simulink model "Two_Input_Model_CO"  (R2021a)
settings: Solver=VariableStepAuto  StartTime=0.0  StopTime=10  RelTol=1e-3
values from neighbouring files (symbols this model uses):
  A = [0 0 0 0 0 0 0 0 0 -0.534142885228 22.5045950602 -13.9882516442 ... (36 elements, 6x6)]    [Values_Rev3.mat]
  B = [0 0 0 0.425188099574 -0.174236211288 -0.288671680413 0 0 0 -0.174236211288 7.34094843962 -4.56293631615 ... (18 elements, 6x3)]    [Values_Rev3.mat]
  C = [1 0 0 0 1 0 0 0 1 0 0 0 ... (18 elements, 3x6)]    [Values_Rev3.mat]
undefined symbols (not defined in the file or in its folder): K, L, v, x0
libraries: vrlib x2, aerolibanimutils x1, dspvision x1
settings Model: Creator=J44381  LastModifiedBy=vicen
settings SolverCC: AlgebraicLoopSolver=TrustRegion
settings DebuggingCC: SFMachineParentedDataDiag=warning

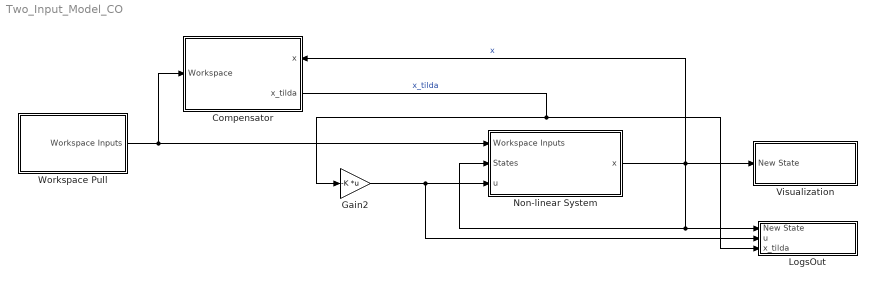
== system Two_Input_Model_CO ==
  Compensator : Subsystem
      settings: PortSchema="{\"entries\":[{\"content\":{\"sides\":[{\"content\":{\"connectorIds\":[\"In1\"]},\"type\":\"ConnectorPlacement.EquallySpacedRectSide\",\"uuid\":\"fa5a8305-86ae-432c-9810-dcf02cae709e\"},{\"content\":{\"connectorIds\":[\"In2\",\"Out1\"],\"side\":\"RIGHT\"},\"type\":\"ConnectorPlacement.EquallySpacedRectSide\",\"uuid\":\"5b9e218f-8372-497e-90c9-36ba94e4ea20\"},{\"content\":{\"connectorIds\":[],\"side\":\"TOP\"},\"type\":\"ConnectorPlacement.EquallySpacedRectSide\",\"uuid\":\"bf766896-0790-4646-8f59-54f411e82d6d\"}]},\"type\":\"ConnectorPlacement.EquallySpacedConnector\",\"uuid\":\"810fb74e-5609-4dc4-a3e8-0485af32c7e5\"}],\"packageUris\":[\"http://schema.mathworks.com/mf0/Connector/R2020b\"],\"version\":\"1.0\"}"
  Gain2 : Gain  Gain=-K  Multiplication=Matrix(K*u)
  LogsOut : Subsystem
  Non-linear System : Subsystem
  Visualization : Subsystem
  Workspace Pull : Subsystem
  wires:
  Workspace Pull/1("Workspace Inputs ") -> Compensator/1(Workspace), Non-linear System/1("Workspace Inputs ")
  Non-linear System/1(x) -> Compensator/2(x), Visualization/1(New State), Non-linear System/2(States), LogsOut/1(New State)  "x"
  Compensator/1(x_tilda) -> Gain2/1, LogsOut/3(x_tilda)  "x_tilda"
  Gain2/1 -> Non-linear System/3(u), LogsOut/2(u)

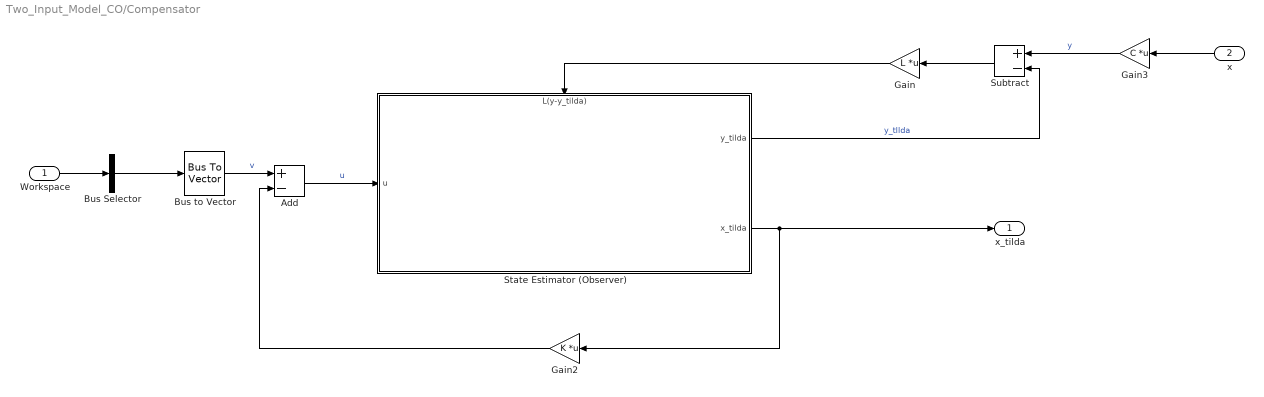
== system Two_Input_Model_CO/Compensator ==
  Workspace : Inport
  x : Inport  Port=2
  Add : Sum  Inputs=+-
  Bus Selector : BusSelector  OutputSignals=Reference_Signal  OutputAsBus=on
  Bus to Vector : BusToVector
  Gain : Gain  Gain=L  Multiplication=Matrix(K*u)
  Gain2 : Gain  Gain=K  Multiplication=Matrix(K*u)
  Gain3 : Gain  Gain=C  Multiplication=Matrix(K*u)
  State Estimator (Observer) : Subsystem
      settings: PortSchema="{\"entries\":[{\"content\":{\"sides\":[{\"content\":{\"connectorIds\":[\"In1\"]},\"type\":\"ConnectorPlacement.EquallySpacedRectSide\",\"uuid\":\"af437ed9-8515-47ce-9bf3-57578eb1cf2e\"},{\"content\":{\"connectorIds\":[\"Out1\",\"Out2\"],\"side\":\"RIGHT\"},\"type\":\"ConnectorPlacement.EquallySpacedRectSide\",\"uuid\":\"1ea6d729-9487-4493-ae4f-2f3f5c430ca0\"},{\"content\":{\"connectorIds\":[\"In2\"],\"side\":\"TOP\"},\"type\":\"ConnectorPlacement.EquallySpacedRectSide\",\"uuid\":\"e9fc0f2c-a064-4175-9528-0d44140d355b\"}]},\"type\":\"ConnectorPlacement.EquallySpacedConnector\",\"uuid\":\"af498723-3483-4ae8-9449-73d3fe9ce68c\"}],\"packageUris\":[\"http://schema.mathworks.com/mf0/Connector/R2020b\"],\"version\":\"1.0\"}"
  Subtract : Sum  Inputs=+-
  x_tilda : Outport
  wires:
  Add/1 -> State Estimator (Observer)/1(u)  "u"
  State Estimator (Observer)/1(y_tilda) -> Subtract/2  "y_tllda"
  Subtract/1 -> Gain/1
  Workspace/1 -> Bus Selector/1
  Bus Selector/1 -> Bus to Vector/1
  Bus to Vector/1 -> Add/1  "v"
  State Estimator (Observer)/2(x_tilda) -> Gain2/1, x_tilda/1
  Gain/1 -> State Estimator (Observer)/2(L(y-y_tilda))
  x/1 -> Gain3/1
  Gain2/1 -> Add/2
  Gain3/1 -> Subtract/1  "y"

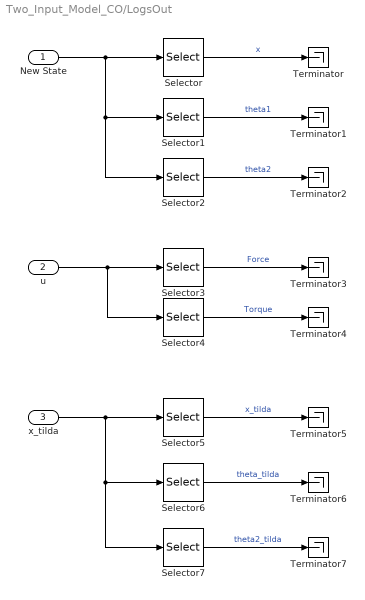
== system Two_Input_Model_CO/LogsOut ==
  New State : Inport
  u : Inport  Port=2
  x_tilda : Inport  Port=3
  Selector : Selector  InputPortWidth=6  IndexOptions=Index vector (dialog)  Indices=1  OutputSizes=1
  Selector1 : Selector  InputPortWidth=6  IndexOptions=Index vector (dialog)  Indices=2  OutputSizes=1
  Selector2 : Selector  InputPortWidth=6  IndexOptions=Index vector (dialog)  Indices=3  OutputSizes=1
  Selector3 : Selector  InputPortWidth=2  IndexOptions=Index vector (dialog)  Indices=1  OutputSizes=1
  Selector4 : Selector  InputPortWidth=2  IndexOptions=Index vector (dialog)  Indices=2  OutputSizes=1
  Selector5 : Selector  InputPortWidth=6  IndexOptions=Index vector (dialog)  Indices=1  OutputSizes=1
  Selector6 : Selector  InputPortWidth=6  IndexOptions=Index vector (dialog)  Indices=2  OutputSizes=1
  Selector7 : Selector  InputPortWidth=6  IndexOptions=Index vector (dialog)  Indices=3  OutputSizes=1
  Terminator{,1..7} (8 alike) : Terminator
  wires:
  Selector/1 -> Terminator/1  "x"
  Selector1/1 -> Terminator1/1  "theta1"
  Selector2/1 -> Terminator2/1  "theta2"
  New State/1 -> Selector2/1, Selector1/1, Selector/1
  u/1 -> Selector4/1, Selector3/1
  Selector4/1 -> Terminator4/1  "Torque"
  Selector3/1 -> Terminator3/1  "Force"
  x_tilda/1 -> Selector5/1, Selector7/1, Selector6/1
  Selector5/1 -> Terminator5/1  "x_tilda"
  Selector6/1 -> Terminator6/1  "theta_tilda"
  Selector7/1 -> Terminator7/1  "theta2_tilda"

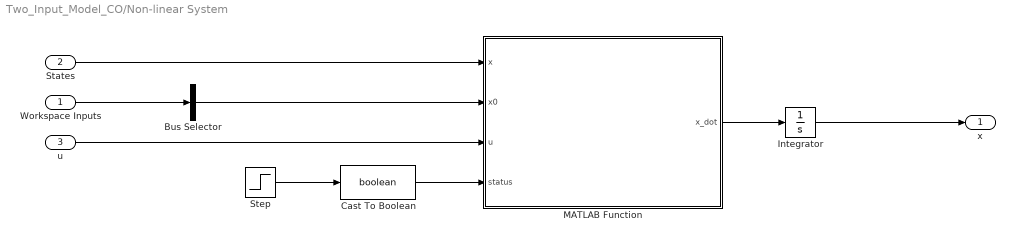
== system Two_Input_Model_CO/Non-linear System ==
  "Workspace Inputs " : Inport
  States : Inport  Port=2
  u : Inport  Port=3
  Bus Selector : BusSelector  OutputSignals=Initial_States  OutputAsBus=on
  Cast To Boolean : DataTypeConversion  OutDataTypeStr=boolean
  Integrator : Integrator  InitialCondition=[x0.x;x0.theta1;x0.theta2;x0.x_dot;x0.theta1_dot;x0.theta2_dot]
  MATLAB Function : MATLAB Function  TreatAsAtomicUnit=on
  Step : Step  Time=.01  SampleTime=0
  x : Outport
  wires:
  MATLAB Function/1(x_dot) -> Integrator/1
  States/1 -> MATLAB Function/1(x)
  "Workspace Inputs "/1 -> Bus Selector/1
  u/1 -> MATLAB Function/3(u)
  Bus Selector/1 -> MATLAB Function/2(x0)
  Integrator/1 -> x/1
  Step/1 -> Cast To Boolean/1
  Cast To Boolean/1 -> MATLAB Function/4(status)

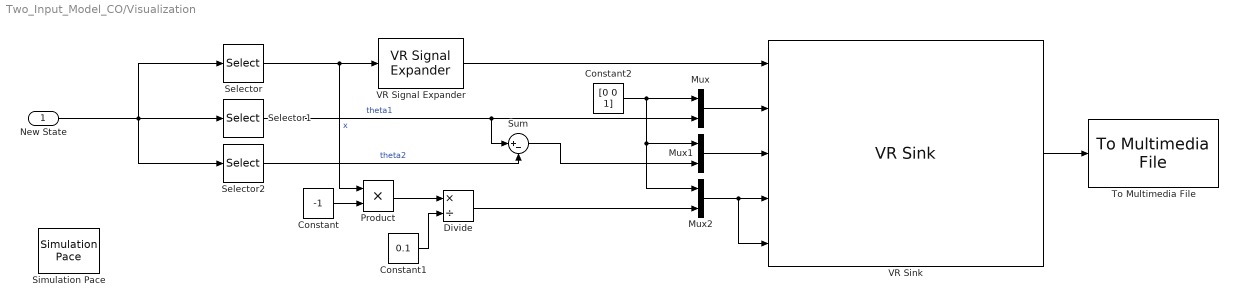
== system Two_Input_Model_CO/Visualization ==
  New State : Inport
  Constant : Constant  Value=-1
  Constant1 : Constant  Value=0.1
  Constant2 : Constant  Value=[0 0 1]
  Divide : Product  Inputs=*/
  Mux : Mux  Inputs=2
  Mux1 : Mux  Inputs=2
  Mux2 : Mux  Inputs=2
  Product : Product
  Selector : Selector  InputPortWidth=6  IndexOptions=Index vector (dialog)  Indices=1  OutputSizes=1
  Selector1 : Selector  InputPortWidth=6  IndexOptions=Index vector (dialog)  Indices=2  OutputSizes=1
  Selector2 : Selector  InputPortWidth=6  IndexOptions=Index vector (dialog)  Indices=3  OutputSizes=1
  Simulation Pace : aerolibanimutils/Simulation Pace  SimulationPace=1  SleepMode=Auto  OutputPaceError=off  SampleTime=1/30
  Sum : Sum  Inputs=|+-
  To Multimedia File : dspvision/To Multimedia File  outputFilename=output2.avi  streamSelection=Video only  videoCompressor=None (uncompressed)  audioCompressor=None (uncompressed)  imagePorts=One multidimensional signal  fileType=AVI  audioDatatype=Determine from input data type  fourcc=RGB  videoQuality=75  mj2000CompFactor=10
  VR Signal Expander : vrlib/VR Signal Expander  outwidth=3  outidx=[1]
  VR Sink : vrlib/VR Sink  InstantiateOnLoad=on  SampleTime=0.1  ViewEnable=on  RemoteChange=off  RemoteView=off  FieldsWritten=Cart.translation.3.1.1.double#Rotation1.rotation.4.1.1.double#Rotation2.rotation.4.1.1.double#Axis_Rotate.rotation.4.1.1.double#Axis_Rotate2.rotation.4.1.1.double  WorldFileName=Cart_Actual.WRL  AutoView=off  VideoDimensions=[1500 2000]  AllowVariableSize=off  FigureProperties="{'Position', 'Name', 'Viewpoint', 'CameraBound', 'CameraDirection', 'CameraPosition', 'CameraUpVector', 'ZoomFactor', 'Antialiasing', 'Headlight', 'Lighting', 'NavPanel', 'Sound', 'StatusBar', 'Stereo3D', 'Stereo3DCameraOffset', 'Stereo3DHIT', 'ToolBar', 'Textures', 'Transparency', 'Triad', 'Wireframe', 'NavZones', 'NavMode', 'NavSpeed', 'CaptureFileFormat', 'CaptureFileName', 'Record2DCompressMethod', 'Record2DCompressQuality', 'Record2D', 'Record2DFileName', 'Record2DFPS'; [1.2660000000000001e+02   9.4799999999999955e+01   8.0000000000000000e+02   6.0020000000000005e+02], '', '_untitled_1', 'on', [0.0000000000000000e+00   0.0000000000000000e+00  -1.0000000000000000e+00], [0.0000000000000000e+00   0.0000000000000000e+00   0.0000000000000000e+00], [0.0000000000000000e+00   1.0000000000000000e+00   0.0000000000000000e+00], [1.0000000000000000e+00], 'on', 'on', 'on', 'none', 'on', 'off', 'off', [1.0000000149011612e-01], [0.0000000000000000e+00], 'off', 'on', 'on', 'none', 'off', 'off', 'fly', 'normal', 'tif', '%f_anim_%n.tif', 'auto', [7.5000000000000000e+01], 'off', '***video***', 'auto'}"
  wires:
  New State/1 -> Selector/1, Selector2/1, Selector1/1
  Selector/1 -> VR Signal Expander/1, Product/1  "x"
  Selector1/1 -> Sum/1, Mux/2  "theta1"
  Product/1 -> Divide/1
  Constant/1 -> Product/2
  Constant1/1 -> Divide/2
  Constant2/1 -> Mux1/1, Mux2/1, Mux/1
  Selector2/1 -> Sum/2  "theta2"
  Divide/1 -> Mux2/2
  Sum/1 -> Mux1/2
  VR Signal Expander/1 -> VR Sink/1
  Mux/1 -> VR Sink/2
  Mux1/1 -> VR Sink/3
  Mux2/1 -> VR Sink/4, VR Sink/5
  VR Sink/1 -> To Multimedia File/1

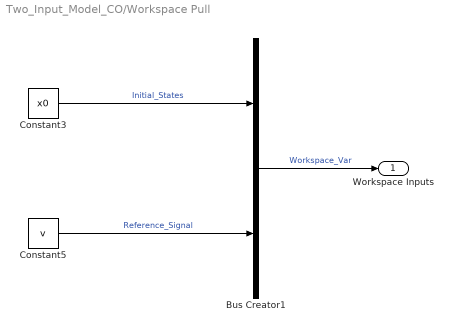
== system Two_Input_Model_CO/Workspace Pull ==
  Bus Creator1 : BusCreator  Inputs=2
  Constant3 : Constant  Value=x0  VectorParams1D=off  OutDataTypeStr=Bus: State_bus
  Constant5 : Constant  Value=v  VectorParams1D=off  OutDataTypeStr=Bus: Reference_bus
  "Workspace Inputs " : Outport
  wires:
  Bus Creator1/1 -> "Workspace Inputs "/1  "Workspace_Var"
  Constant3/1 -> Bus Creator1/1  "Initial_States"
  Constant5/1 -> Bus Creator1/2  "Reference_Signal"

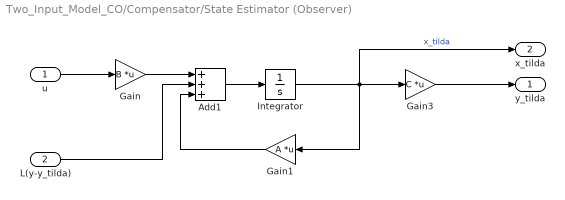
== system Two_Input_Model_CO/Compensator/State Estimator (Observer) ==
  u : Inport
  L(y-y_tilda) : Inport  Port=2
  Add1 : Sum  Inputs=+++
  Gain : Gain  Gain=B  Multiplication=Matrix(K*u)
  Gain1 : Gain  Gain=A  Multiplication=Matrix(K*u)
  Gain3 : Gain  Gain=C  Multiplication=Matrix(K*u)
  Integrator : Integrator  InitialCondition=[x0.x;0;0;x0.x_dot;x0.theta1_dot;x0.theta2_dot]
  y_tilda : Outport
  x_tilda : Outport  Port=2
  wires:
  Gain1/1 -> Add1/3
  Integrator/1 -> Gain3/1, x_tilda/1, Gain1/1  "x_tilda"
  Add1/1 -> Integrator/1
  Gain/1 -> Add1/1
  u/1 -> Gain/1
  Gain3/1 -> y_tilda/1
  L(y-y_tilda)/1 -> Add1/2

== matlab function Two_Input_Model_CO/Non-linear System/MATLAB Function ==
  data: x input; x0 input; u input; x_dot output; status input
function x_dot  = Nonlinear_Dynamics(x,x0,u,status)
    if status == false
        x2 = x0.theta1;
        x3 = x0.theta2;
        x4 = x0.x_dot;
        x5 = x0.theta1_dot;
        x6 = x0.theta2_dot;
        u1 = u(1);
        u2 = u(2);
    else
        x2 = x(2);
        x3 = x(3);
        x4 = x(4);
        x5 = x(5);
        x6 = x(6);
        u1 = u(1);
        u2 = u(2);
    end
    % Insert Equations
    x_dot = double([
                x4;
                x5;
                x6;
                x5*((15*x5*sin(x2 - x3)*(cos(x3) - cos(x2 - x3)*cos(x2)))/(2*(25*cos(x2)^2 + 15*cos(x3)^2 + 33*cos(x2 - x3)^2 - 30*cos(x2 - x3)*cos(x2)*cos(x3) - 55)) + (5*x5*sin(x2)*(3*cos(x2 - x3)^2 - 5))/(2*(25*cos(x2)^2 + 15*cos(x3)^2 + 33*cos(x2 - x3)^2 - 30*cos(x2 - x3)*cos(x2)*cos(x3) - 55))) - x6*((9*x6*sin(x2 - x3)*(5*cos(x2) - 3*cos(x2 - x3)*cos(x3)))/(4*(25*cos(x2)^2 + 15*cos(x3)^2 + 33*cos(x2 - x3)^2 - 30*cos(x2 - x3)*cos(x2)*cos(x3) - 55)) - (9*x6*sin(x3)*(3*cos(x2 - x3)^2 - 5))/(4*(25*cos(x2)^2 + 15*cos(x3)^2 + 33*cos(x2 - x3)^2 - 30*cos(x2 - x3)*cos(x2)*cos(x3) - 55))) + (981*sin(x2)*(5*cos(x2) - 3*cos(x2 - x3)*cos(x3)))/(20*(25*cos(x2)^2 + 15*cos(x3)^2 + 33*cos(x2 - x3)^2 - 30*cos(x2 - x3)*cos(x2)*cos(x3) - 55)) + (8*u2*(5*cos(x2) - 3*cos(x2 - x3)*cos(x3)))/(25*cos(x2)^2 + 15*cos(x3)^2 + 33*cos(x2 - x3)^2 - 30*cos(x2 - x3)*cos(x2)*cos(x3) - 55) + (2943*sin(x3)*(cos(x3) - cos(x2 - x3)*cos(x2)))/(20*(25*cos(x2)^2 + 15*cos(x3)^2 + 33*cos(x2 - x3)^2 - 30*cos(x2 - x3)*cos(x2)*cos(x3) - 55)) + (4*u1*(3*cos(x2 - x3)^2 - 5))/(25*cos(x2)^2 + 15*cos(x3)^2 + 33*cos(x2 - x3)^2 - 30*cos(x2 - x3)*cos(x2)*cos(x3) - 55);
                x5*((5*x5*sin(x2)*(5*cos(x2) - 3*cos(x2 - x3)*cos(x3)))/(25*cos(x2)^2 + 15*cos(x3)^2 + 33*cos(x2 - x3)^2 - 30*cos(x2 - x3)*cos(x2)*cos(x3) - 55) + (3*x5*sin(x2 - x3)*(11*cos(x2 - x3) - 5*cos(x2)*cos(x3)))/(25*cos(x2)^2 + 15*cos(x3)^2 + 33*cos(x2 - x3)^2 - 30*cos(x2 - x3)*cos(x2)*cos(x3) - 55)) + x6*((9*x6*sin(x3)*(5*cos(x2) - 3*cos(x2 - x3)*cos(x3)))/(2*(25*cos(x2)^2 + 15*cos(x3)^2 + 33*cos(x2 - x3)^2 - 30*cos(x2 - x3)*cos(x2)*cos(x3) - 55)) - (9*x6*sin(x2 - x3)*(3*cos(x3)^2 - 11))/(2*(25*cos(x2)^2 + 15*cos(x3)^2 + 33*cos(x2 - x3)^2 - 30*cos(x2 - x3)*cos(x2)*cos(x3) - 55))) + (2943*sin(x3)*(11*cos(x2 - x3) - 5*cos(x2)*cos(x3)))/(50*(25*cos(x2)^2 + 15*cos(x3)^2 + 33*cos(x2 - x3)^2 - 30*cos(x2 - x3)*cos(x2)*cos(x3) - 55)) + (981*sin(x2)*(3*cos(x3)^2 - 11))/(10*(25*cos(x2)^2 + 15*cos(x3)^2 + 33*cos(x2 - x3)^2 - 30*cos(x2 - x3)*cos(x2)*cos(x3) - 55)) + (8*u1*(5*cos(x2) - 3*cos(x2 - x3)*cos(x3)))/(25*cos(x2)^2 + 15*cos(x3)^2 + 33*cos(x2 - x3)^2 - 30*cos(x2 - x3)*cos(x2)*cos(x3) - 55) + (16*u2*(3*cos(x3)^2 - 11))/(25*cos(x2)^2 + 15*cos(x3)^2 + 33*cos(x2 - x3)^2 - 30*cos(x2 - x3)*cos(x2)*cos(x3) - 55);
                x6*((15*x6*sin(x3)*(cos(x3) - cos(x2 - x3)*cos(x2)))/(25*cos(x2)^2 + 15*cos(x3)^2 + 33*cos(x2 - x3)^2 - 30*cos(x2 - x3)*cos(x2)*cos(x3) - 55) - (3*x6*sin(x2 - x3)*(11*cos(x2 - x3) - 5*cos(x2)*cos(x3)))/(25*cos(x2)^2 + 15*cos(x3)^2 + 33*cos(x2 - x3)^2 - 30*cos(x2 - x3)*cos(x2)*cos(x3) - 55)) + x5*((50*x5*sin(x2)*(cos(x3) - cos(x2 - x3)*cos(x2)))/(3*(25*cos(x2)^2 + 15*cos(x3)^2 + 33*cos(x2 - x3)^2 - 30*cos(x2 - x3)*cos(x2)*cos(x3) - 55)) + (10*x5*sin(x2 - x3)*(5*cos(x2)^2 - 11))/(3*(25*cos(x2)^2 + 15*cos(x3)^2 + 33*cos(x2 - x3)^2 - 30*cos(x2 - x3)*cos(x2)*cos(x3) - 55))) + (327*sin(x2)*(11*cos(x2 - x3) - 5*cos(x2)*cos(x3)))/(5*(25*cos(x2)^2 + 15*cos(x3)^2 + 33*cos(x2 - x3)^2 - 30*cos(x2 - x3)*cos(x2)*cos(x3) - 55)) + (327*sin(x3)*(5*cos(x2)^2 - 11))/(5*(25*cos(x2)^2 + 15*cos(x3)^2 + 33*cos(x2 - x3)^2 - 30*cos(x2 - x3)*cos(x2)*cos(x3) - 55)) + (80*u1*(cos(x3) - cos(x2 - x3)*cos(x2)))/(3*(25*cos(x2)^2 + 15*cos(x3)^2 + 33*cos(x2 - x3)^2 - 30*cos(x2 - x3)*cos(x2)*cos(x3) - 55)) + (32*u2*(11*cos(x2 - x3) - 5*cos(x2)*cos(x3)))/(3*(25*cos(x2)^2 + 15*cos(x3)^2 + 33*cos(x2 - x3)^2 - 30*cos(x2 - x3)*cos(x2)*cos(x3) - 55))]);
 
end
